simulink model "VehicleEnergyManagementSystem"  (R2024b)
settings: Solver=VariableStepAuto  StartTime=0.0  StopTime=150  RelTol=1e-3
InitFcn:
  | run("MPC\Initialization.m")
model workspace (MAT data in the model file):
  MotorTorqueMax = 500
  WheelRadius = 0.3
values from neighbouring files (symbols this model uses):
  motorBackEMFConstant = 0.004    [GenerateDiscretizedModels.m]    (also in Initialization.m)
  motorInductance = 0.005    [GenerateDiscretizedModels.m]    (also in Initialization.m)
  motorResistance = 0.1    [GenerateDiscretizedModels.m]    (also in Initialization.m)
  motorTorqueConstant = 5    [GenerateDiscretizedModels.m]    (also in Initialization.m)
undefined symbols (not defined in the file or in its folder): InputWeightMatrix, SelectedRoadCoefficients, StateWeightMatrix
libraries: MultiModelToolbox x6, autolibshared x6
(part 2 of 2)

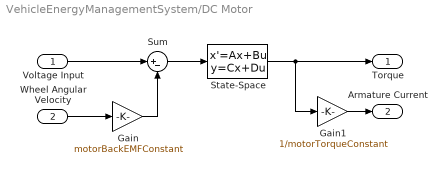
== system VehicleEnergyManagementSystem/DC Motor ==
  Voltage Input : Inport
  Wheel Angular Velocity : Inport  Port=2
  Gain : Gain  Gain=motorBackEMFConstant
  Gain1 : Gain  Gain=1/motorTorqueConstant
  State-Space : StateSpace  A=-motorResistance/motorInductance  B=1/motorInductance  C=motorTorqueConstant  D=0  InitialCondition=0
  Sum : Sum  Inputs=|+-
  Torque : Outport
  Armature Current : Outport  Port=2
  wires:
  Voltage Input/1 -> Sum/1
  Gain/1 -> Sum/2
  Wheel Angular Velocity/1 -> Gain/1
  Sum/1 -> State-Space/1
  State-Space/1 -> Torque/1, Gain1/1
  Gain1/1 -> Armature Current/1

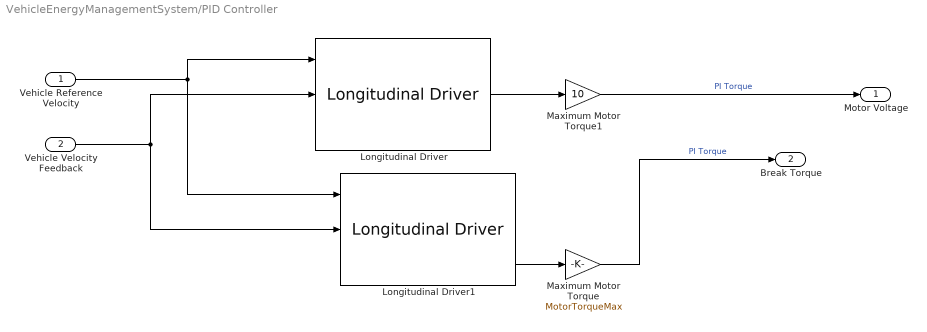
== system VehicleEnergyManagementSystem/PID Controller ==
  Vehicle Reference Velocity : Inport
  Vehicle Velocity Feedback : Inport  Port=2
  Longitudinal Driver : autolibshared/Longitudinal Driver  extAccelOvr=off  extDecelOvr=off  extAccelHld=off  extDecelHld=off  extAccelZero=off  extDecelZero=off  cntrlType=PI  shftType=None  velUnits=m/s  gearOut=off  Kp=3  Ki=1  Kff=.1  Kg=0  VehVelVec=[0 100]  KffVec=[.1 .1]  KpVec=[10 10]  KiVec=[5 5]  KgVec=[0 0]  m=1500  Kpt=3000  tau=.1  L=2  aR=200  bR=2.5  cR=.5  g=9.81  vnom=5  Kaw=1  tauerr=.01  tauPt=2  GearInit=0  tShift=.1  pdlVec=[0.1 0.4 0.5 0.9]  upShftTbl=[-1 12.9375 26.4375 39.9375 51.18749999999999 62.4375 72.84375 83.25;-1 16.3125 29.8125 43.3125 54.5624 65.8125 76.78125 87.75;-1 19.6875 33.1875 46.68749999999999 57.9375 69.1875 80.71875 92.25;-1 33 52.5 77.25 100.5 138.75 161.875 185]  dwnShftTbl=[1 9.5625 23.0625 36.5625 47.8125 59.0625 68.90625 78.75;1 12.9375 26.4375 39.9375 51.18749999999999 62.4375 72.84375 83.25;1 16.3125 29.8125 43.3125 54.562499 65.8125 76.78125 87.75;1 19.6875 33.1875 46.68749999999999 57.9375 69.1875 80.71875 92.25]  tClutch=.5  tRev=.5  tPark=120  aMode=2  UpGearVec="[0  1  2  3  4  5  6  7]"  DownGearVec="[1  2  3  4  5  6  7  8]"
      settings: LibrarySourceBlock=vehdynlibdriver/Longitudinal Driver
  Longitudinal Driver1 : autolibshared/Longitudinal Driver  extAccelOvr=off  extDecelOvr=off  extAccelHld=off  extDecelHld=off  extAccelZero=off  extDecelZero=off  cntrlType=PI  shftType=None  velUnits=m/s  gearOut=off  Kp=8  Ki=2  Kff=.1  Kg=0  VehVelVec=[0 100]  KffVec=[.1 .1]  KpVec=[10 10]  KiVec=[5 5]  KgVec=[0 0]  m=1500  Kpt=3000  tau=.1  L=2  aR=200  bR=2.5  cR=.5  g=9.81  vnom=5  Kaw=1  tauerr=.01  tauPt=2  GearInit=0  tShift=.1  pdlVec=[0.1 0.4 0.5 0.9]  upShftTbl=[-1 12.9375 26.4375 39.9375 51.18749999999999 62.4375 72.84375 83.25;-1 16.3125 29.8125 43.3125 54.5624 65.8125 76.78125 87.75;-1 19.6875 33.1875 46.68749999999999 57.9375 69.1875 80.71875 92.25;-1 33 52.5 77.25 100.5 138.75 161.875 185]  dwnShftTbl=[1 9.5625 23.0625 36.5625 47.8125 59.0625 68.90625 78.75;1 12.9375 26.4375 39.9375 51.18749999999999 62.4375 72.84375 83.25;1 16.3125 29.8125 43.3125 54.562499 65.8125 76.78125 87.75;1 19.6875 33.1875 46.68749999999999 57.9375 69.1875 80.71875 92.25]  tClutch=.5  tRev=.5  tPark=120  aMode=2  UpGearVec="[0  1  2  3  4  5  6  7]"  DownGearVec="[1  2  3  4  5  6  7  8]"
      settings: LibrarySourceBlock=vehdynlibdriver/Longitudinal Driver
  Maximum Motor Torque : Gain  Gain=MotorTorqueMax
  Maximum Motor Torque1 : Gain  Gain=10
  Motor Voltage : Outport
  Break Torque : Outport  Port=2
  wires:
  Longitudinal Driver/2 -> Maximum Motor Torque1/1
  Longitudinal Driver1/3 -> Maximum Motor Torque/1
  Vehicle Reference Velocity/1 -> Longitudinal Driver/1, Longitudinal Driver1/1
  Vehicle Velocity Feedback/1 -> Longitudinal Driver/2, Longitudinal Driver1/2
  Maximum Motor Torque/1 -> Break Torque/1  "PI Torque"
  Maximum Motor Torque1/1 -> Motor Voltage/1  "PI Torque"
